simulink model "SWC_HALIN_CDD_type"  (R2021b)
settings: Solver=FixedStepDiscrete  StartTime=0.0  StopTime=10.0  FixedStep=0.005  RelTol=1e-3
undefined symbols (not defined in the file or in its folder): C_TASK_5MS_S, DIDLen_APSFunConfig, DIDLen_AutoLock, DIDLen_AutoWipHSpdEN, DIDLen_DKCKey, DIDLen_DRLDis, DIDLen_DynoMode, DIDLen_FMHTimer, DIDLen_OBDReq, DIDLen_TestGroup, DIDLen_TireSize, DIDLen_TurnLampFLThreCurr, DIDLen_TurnLampFRThreCurr, DIDLen_TurnLampRLThreCurr, DIDLen_TurnLampRRThreCurr, DIDLen_USSConfig, DIDLen_WipRLSCmdCutFilter, DIDLen_WipRLSCmdHoldFilter, DIDLen_XWDMode, DIDNum_APSFunConfig, DIDNum_AutoLock, DIDNum_AutoWipHSpdEN, DIDNum_DKCKey, DIDNum_DRLDis, DIDNum_DynoMode, DIDNum_FMHTimer, DIDNum_OBDReq, DIDNum_TestGroup, DIDNum_TireSize, DIDNum_TurnLampFLThreCurr, DIDNum_TurnLampFRThreCurr, DIDNum_TurnLampRLThreCurr, DIDNum_TurnLampRRThreCurr, DIDNum_USSConfig, DIDNum_WipRLSCmdCutFilter, DIDNum_WipRLSCmdHoldFilter, DIDNum_XWDMode, ENUM_DRIVETRAIN_AWD, ENUM_DRIVETRAIN_FWD, ENUM_DRIVETRAIN_RWD, ENUM_REGENLEVEL_LV1, ENUM_REGENLEVEL_LV2, ENUM_REGENLEVEL_LV3, ENUM_REGENLEVEL_LV4, ENUM_REGENLEVEL_LV5, ENUM_REGENLEVEL_OPD, ENUM_TPMSSTA_FAT, ENUM_TPMSSTA_LOWBATTERY, ENUM_TPMSSTA_TRIGGER, FALSE, FIVE_INT, FOUR_INT, KHAL_CANBusOffDebounce_s, KHAL_DefaultRegenMode_enum, KHAL_DKCDecryptEnable_flg_ovrdflg, KHAL_DKCDecryptEnable_flg_ovrdval, KHAL_RandomNumberY1_enum, KHAL_RandomNumberY2_enum, KHAL_RandomNumberY_ovrdflg, KHAL_TPMSRESBUTT_flg_ovrdflg ... (+9)
libraries: simulink x229, FVT_lib x29, hcu_lib x25, hdlsllib x15
(part 2 of 8)

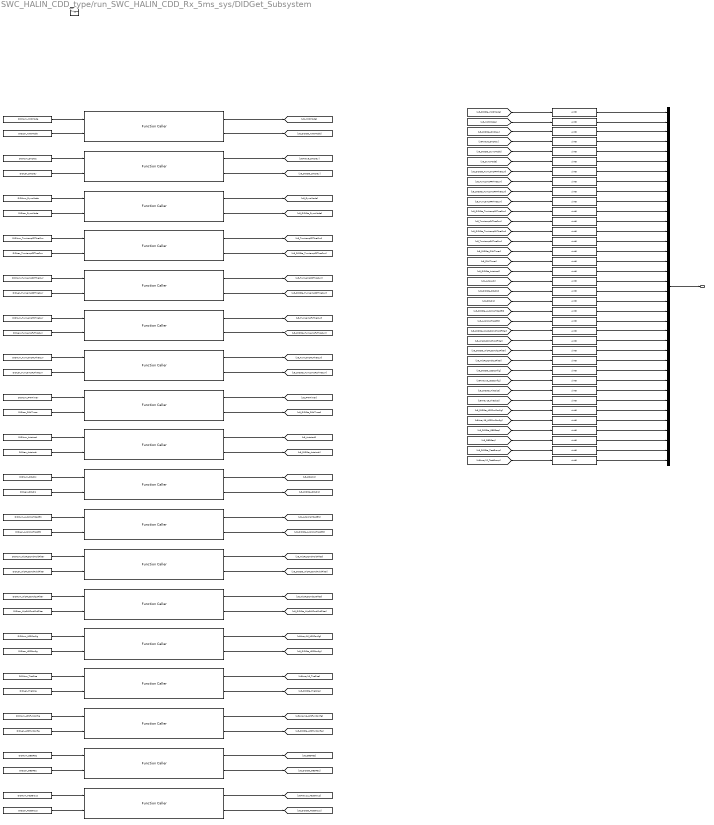
== system SWC_HALIN_CDD_type/run_SWC_HALIN_CDD_Rx_5ms_sys/DIDGet_Subsystem ==
  trig_GetDID : TriggerPort  TriggerType=function-call  VariantControl=(inherit)  PortDimensions=1
  DIDLen : Constant  Value=DIDNum_XWDMode
  DIDLen1 : Constant  Value=DIDNum_DKCKey
  DIDLen10 : Constant  Value=DIDNum_AutoWipHSpdEN
  DIDLen11 : Constant  Value=DIDNum_WipRLSCmdHoldFilter
  DIDLen12 : Constant  Value=DIDNum_WipRLSCmdCutFilter
  DIDLen13 : Constant  Value=DIDNum_USSConfig
  DIDLen14 : Constant  Value=DIDNum_TireSize
  DIDLen15 : Constant  Value=DIDNum_APSFunConfig
  DIDLen16 : Constant  Value=DIDNum_OBDReq
  DIDLen17 : Constant  Value=DIDNum_TestGroup
  DIDLen2 : Constant  Value=DIDNum_DynoMode
  DIDLen3 : Constant  Value=DIDNum_TurnLampFRThreCurr
  DIDLen4 : Constant  Value=DIDNum_TurnLampRRThreCurr
  DIDLen5 : Constant  Value=DIDNum_TurnLampFLThreCurr
  DIDLen6 : Constant  Value=DIDNum_TurnLampRLThreCurr
  DIDLen7 : Constant  Value=DIDNum_FMHTimer
  DIDLen8 : Constant  Value=DIDNum_AutoLock
  DIDLen9 : Constant  Value=DIDNum_DRLDis
  DIDNum : Constant  Value=DIDLen_XWDMode
  DIDNum1 : Constant  Value=DIDLen_DKCKey
  DIDNum10 : Constant  Value=DIDLen_AutoWipHSpdEN
  DIDNum11 : Constant  Value=DIDLen_WipRLSCmdHoldFilter
  DIDNum12 : Constant  Value=DIDLen_WipRLSCmdCutFilter
  DIDNum13 : Constant  Value=DIDLen_USSConfig
  DIDNum14 : Constant  Value=DIDLen_TireSize
  DIDNum15 : Constant  Value=DIDLen_APSFunConfig
  DIDNum16 : Constant  Value=DIDLen_OBDReq
  DIDNum17 : Constant  Value=DIDLen_TestGroup
  DIDNum2 : Constant  Value=DIDLen_DynoMode
  DIDNum3 : Constant  Value=DIDLen_TurnLampFRThreCurr
  DIDNum4 : Constant  Value=DIDLen_TurnLampRRThreCurr
  DIDNum5 : Constant  Value=DIDLen_TurnLampFLThreCurr
  DIDNum6 : Constant  Value=DIDLen_TurnLampRLThreCurr
  DIDNum7 : Constant  Value=DIDLen_FMHTimer
  DIDNum8 : Constant  Value=DIDLen_AutoLock
  DIDNum9 : Constant  Value=DIDLen_DRLDis
  R_DIDReadCDD_CSOP_DIDGet_APSFunConfig : FunctionCaller  FunctionPrototype=[u8Array16_APSFunConfig,u8_DIDSta_APSFunConfig] = R_DIDReadCDD_CSOP_DIDGet_APSFunConfig(u16_DIDNum_APSFunConfig,u16_DIDLen_APSFunConfig)  InputArgumentSpecifications=uint16(1), uint16(1)  OutputArgumentSpecifications=uint8([1;1;1;1;1;1;1;1;1;1;1;1;1;1;1;1]), uint8(1)
  R_DIDReadCDD_CSOP_DIDGet_AutoLock : FunctionCaller  FunctionPrototype=[u8_AutoLock,u8_DIDSta_AutoLock] = R_DIDReadCDD_CSOP_DIDGet_AutoLock(u16_DIDNum_AutoLock,u16_DIDLen_AutoLock)  InputArgumentSpecifications=uint16(1), uint16(1)  OutputArgumentSpecifications=uint8(1), uint8(1)
  R_DIDReadCDD_CSOP_DIDGet_AutoWipHSpdEN : FunctionCaller  FunctionPrototype=[u8_AutoWipHSpdEN,u8_DIDSta_AutoWipHSpdEN] = R_DIDReadCDD_CSOP_DIDGet_AutoWipHSpdEN(u16_DIDNum_AutoWipHSpdEN,u16_DIDLen_AutoWipHSpdEN)  InputArgumentSpecifications=uint16(1), uint16(1)  OutputArgumentSpecifications=uint8(1), uint8(1)
  R_DIDReadCDD_CSOP_DIDGet_DKCKey : FunctionCaller  FunctionPrototype=[u8Array8_DKCKey,u8_DIDSta_DKCKey] = R_DIDReadCDD_CSOP_DIDGet_DKCKey(u16_DIDNum_DKCKey,u16_DIDLen_DKCKey)  InputArgumentSpecifications=uint16(1), uint16(1)  OutputArgumentSpecifications=uint8([1;1;1;1;1;1;1;1]), uint8(1)
  R_DIDReadCDD_CSOP_DIDGet_DRLDis : FunctionCaller  FunctionPrototype=[u8_DRLDis,u8_DIDSta_DRLDis] = R_DIDReadCDD_CSOP_DIDGet_DRLDis(u16_DIDNum_DRLDis,u16_DIDLen_DRLDis)  InputArgumentSpecifications=uint16(1), uint16(1)  OutputArgumentSpecifications=uint8(1), uint8(1)
  R_DIDReadCDD_CSOP_DIDGet_DynoMode : FunctionCaller  FunctionPrototype=[u8_DynoMode,u8_DIDSta_DynoMode] = R_DIDReadCDD_CSOP_DIDGet_DynoMode(u16_DIDNum_DynoMode,u16_DIDLen_DynoMode)  InputArgumentSpecifications=uint16(1), uint16(1)  OutputArgumentSpecifications=uint8(1), uint8(1)
  R_DIDReadCDD_CSOP_DIDGet_FMHTimer : FunctionCaller  FunctionPrototype=[u8_FMHTimer,u8_DIDSta_FMHTimer] = R_DIDReadCDD_CSOP_DIDGet_FMHTimer(u16_DIDNum_FMHTimer,u16_DIDLen_FMHTimer)  InputArgumentSpecifications=uint16(1), uint16(1)  OutputArgumentSpecifications=uint8(1), uint8(1)
  R_DIDReadCDD_CSOP_DIDGet_OBDReq : FunctionCaller  FunctionPrototype=[u8_OBDReq,u8_DIDSta_OBDReq] = R_DIDReadCDD_CSOP_DIDGet_OBDReq(u16_DIDNum_OBDReq,u16_DIDLen_OBDReq)  InputArgumentSpecifications=uint16(1), uint16(1)  OutputArgumentSpecifications=uint8(1), uint8(1)
  R_DIDReadCDD_CSOP_DIDGet_TestGroup : FunctionCaller  FunctionPrototype=[u8Array12_TestGroup,u8_DIDSta_TestGroup] = R_DIDReadCDD_CSOP_DIDGet_TestGroup(u16_DIDNum_TestGroup,u16_DIDLen_TestGroup)  InputArgumentSpecifications=uint16(1), uint16(1)  OutputArgumentSpecifications=uint8([1;1;1;1;1;1;1;1;1;1;1;1]), uint8(1)
  R_DIDReadCDD_CSOP_DIDGet_TireSize : FunctionCaller  FunctionPrototype=[u8Array16_TireSize,u8_DIDSta_TireSize] = R_DIDReadCDD_CSOP_DIDGet_TireSize(u16_DIDNum_TireSize,u16_DIDLen_TireSize)  InputArgumentSpecifications=uint16(1), uint16(1)  OutputArgumentSpecifications=uint8([1;1;1;1;1;1;1;1;1;1;1;1;1;1;1;1]), uint8(1)
  R_DIDReadCDD_CSOP_DIDGet_TurnLampFLThreCurr : FunctionCaller  FunctionPrototype=[u8_TurnLampFLThreCurr,u8_DIDSta_TurnLampFLThreCurr] = R_DIDReadCDD_CSOP_DIDGet_TurnLampFLThreCurr(u16_DIDNum_TurnLampFLThreCurr,u16_DIDLen_TurnLampFLThreCurr)  InputArgumentSpecifications=uint16(1), uint16(1)  OutputArgumentSpecifications=uint8(1), uint8(1)
  R_DIDReadCDD_CSOP_DIDGet_TurnLampFRThreCurr : FunctionCaller  FunctionPrototype=[u8_TurnLampFRThreCurr,u8_DIDSta_TurnLampFRThreCurr] = R_DIDReadCDD_CSOP_DIDGet_TurnLampFRThreCurr(u16_DIDNum_TurnLampFRThreCurr,u16_DIDLen_TurnLampFRThreCurr)  InputArgumentSpecifications=uint16(1), uint16(1)  OutputArgumentSpecifications=uint8(1), uint8(1)
  R_DIDReadCDD_CSOP_DIDGet_TurnLampRLThreCurr : FunctionCaller  FunctionPrototype=[u8_TurnLampRLThreCurr,u8_DIDSta_TurnLampRLThreCurr] = R_DIDReadCDD_CSOP_DIDGet_TurnLampRLThreCurr(u16_DIDNum_TurnLampRLThreCurr,u16_DIDLen_TurnLampRLThreCurr)  InputArgumentSpecifications=uint16(1), uint16(1)  OutputArgumentSpecifications=uint8(1), uint8(1)
  R_DIDReadCDD_CSOP_DIDGet_TurnLampRRThreCurr : FunctionCaller  FunctionPrototype=[u8_TurnLampRRThreCurr,u8_DIDSta_TurnLampRRThreCurr] = R_DIDReadCDD_CSOP_DIDGet_TurnLampRRThreCurr(u16_DIDNum_TurnLampRRThreCurr,u16_DIDLen_TurnLampRRThreCurr)  InputArgumentSpecifications=uint16(1), uint16(1)  OutputArgumentSpecifications=uint8(1), uint8(1)
  R_DIDReadCDD_CSOP_DIDGet_USSConfig : FunctionCaller  FunctionPrototype=[u8Array16_USSConfig,u8_DIDSta_USSConfig] = R_DIDReadCDD_CSOP_DIDGet_USSConfig(u16_DIDNum_USSConfig,u16_DIDLen_USSConfig)  InputArgumentSpecifications=uint16(1), uint16(1)  OutputArgumentSpecifications=uint8([1;1;1;1;1;1;1;1;1;1;1;1;1;1;1;1]), uint8(1)
  R_DIDReadCDD_CSOP_DIDGet_WipRLSCmdCutFilter : FunctionCaller  FunctionPrototype=[u8_WipRLSCmdCutFilter,u8_DIDSta_WipRLSCmdCutFilter] = R_DIDReadCDD_CSOP_DIDGet_WipRLSCmdCutFilter(u16_DIDNum_WipRLSCmdCutFilter,u16_DIDLen_WipRLSCmdCutFilter)  InputArgumentSpecifications=uint16(1), uint16(1)  OutputArgumentSpecifications=uint8(1), uint8(1)
  R_DIDReadCDD_CSOP_DIDGet_WipRLSCmdHoldFilter : FunctionCaller  FunctionPrototype=[u8_WipRLSCmdHoldFilter,u8_DIDSta_WipRLSCmdHoldFilter] = R_DIDReadCDD_CSOP_DIDGet_WipRLSCmdHoldFilter(u16_DIDNum_WipRLSCmdHoldFilter,u16_DIDLen_WipRLSCmdHoldFilter)  InputArgumentSpecifications=uint16(1), uint16(1)  OutputArgumentSpecifications=uint8(1), uint8(1)
  R_DIDReadCDD_CSOP_DIDGet_XWDMode : FunctionCaller  FunctionPrototype=[u8_XWDMode,u8_DIDSta_XWDMode] = R_DIDReadCDD_CSOP_DIDGet_XWDMode(u16_DIDNum_XWDMode,u16_DIDLen_XWDMode)  InputArgumentSpecifications=uint16(1), uint16(1)  OutputArgumentSpecifications=uint8(1), uint8(1)
  UnitConverter{,1..35} (36 alike) : DataTypeConversion  OutDataTypeStr=uint8
  bus_Creator : BusCreator  Inputs=36  OutDataTypeStr=Bus: BHAL_DID_outputs  NonVirtualBus=on
  BHAL_DID_outputs : Outport  OutDataTypeStr=Bus: BHAL_DID_outputs
  wires:
  [u8_DIDSta_XWDMode] -> UnitConverter/1  "u8_DIDSta_XWDMode"
  UnitConverter/1 -> bus_Creator/1  "VHAL_DIDStaXWDMode_raw"
  [u8_XWDMode] -> UnitConverter1/1  "u8_XWDMode"
  UnitConverter1/1 -> bus_Creator/2  "VHAL_XWDMode_raw"
  [u8_DIDSta_DKCKey] -> UnitConverter2/1  "u8_DIDSta_DKCKey"
  UnitConverter2/1 -> bus_Creator/3  "VHAL_DIDStaDKCKey_raw"
  [u8Array8_DKCKey] -> UnitConverter3/1  "u8Array8_DKCKey"
  UnitConverter3/1 -> bus_Creator/4  "VHAL_DKCKey_raw"
  [u8_DIDSta_DynoMode] -> UnitConverter4/1  "u8_DIDSta_DynoMode"
  UnitConverter4/1 -> bus_Creator/5  "VHAL_DIDStaDynoMode_raw"
  [u8_DynoMode] -> UnitConverter5/1  "u8_DynoMode"
  UnitConverter5/1 -> bus_Creator/6  "VHAL_DynoMode_raw"
  [u8_DIDSta_TurnLampFRThreCurr] -> UnitConverter6/1  "u8_DIDSta_TurnLampFRThreCurr"
  UnitConverter6/1 -> bus_Creator/7  "VHAL_DIDStaTurnLampFRThreCurr_raw"
  [u8_TurnLampFRThreCurr] -> UnitConverter7/1  "u8_TurnLampFRThreCurr"
  UnitConverter7/1 -> bus_Creator/8  "VHAL_TurnLampFRThreCurr_raw"
  [u8_DIDSta_TurnLampRRThreCurr] -> UnitConverter8/1  "u8_DIDSta_TurnLampRRThreCurr"
  UnitConverter8/1 -> bus_Creator/9  "VHAL_DIDStaTurnLampRRThreCurr_raw"
  [u8_TurnLampRRThreCurr] -> UnitConverter9/1  "u8_TurnLampRRThreCurr"
  UnitConverter9/1 -> bus_Creator/10  "VHAL_TurnLampRRThreCurr_raw"
  [u8_DIDSta_TurnLampFLThreCurr] -> UnitConverter10/1  "u8_DIDSta_TurnLampFLThreCurr"
  UnitConverter10/1 -> bus_Creator/11  "VHAL_DIDStaTurnLampFLThreCurr_raw"
  [u8_TurnLampFLThreCurr] -> UnitConverter11/1  "u8_TurnLampFLThreCurr"
  UnitConverter11/1 -> bus_Creator/12  "VHAL_TurnLampFLThreCurr_raw"
  [u8_DIDSta_TurnLampRLThreCurr] -> UnitConverter12/1  "u8_DIDSta_TurnLampRLThreCurr"
  UnitConverter12/1 -> bus_Creator/13  "VHAL_DIDStaTurnLampRLThreCurr_raw"
  [u8_TurnLampRLThreCurr] -> UnitConverter13/1  "u8_TurnLampRLThreCurr"
  UnitConverter13/1 -> bus_Creator/14  "VHAL_TurnLampRLThreCurr_raw"
  [u8_DIDSta_FMHTimer] -> UnitConverter14/1  "u8_DIDSta_FMHTimer"
  UnitConverter14/1 -> bus_Creator/15  "VHAL_DIDStaFMHTimer_raw"
  [u8_FMHTimer] -> UnitConverter15/1  "u8_FMHTimer"
  UnitConverter15/1 -> bus_Creator/16  "VHAL_FMHTimer_raw"
  [u8_DIDSta_AutoLock] -> UnitConverter16/1  "u8_DIDSta_AutoLock"
  UnitConverter16/1 -> bus_Creator/17  "VHAL_DIDStaAutoLock_raw"
  [u8_AutoLock] -> UnitConverter17/1  "u8_AutoLock"
  UnitConverter17/1 -> bus_Creator/18  "VHAL_AutoLock_raw"
  [u8_DIDSta_DRLDis] -> UnitConverter18/1  "u8_DIDSta_DRLDis"
  UnitConverter18/1 -> bus_Creator/19  "VHAL_DIDStaDRLDis_raw"
  [u8_DRLDis] -> UnitConverter19/1  "u8_DRLDis"
  UnitConverter19/1 -> bus_Creator/20  "VHAL_DRLDis_raw"
  [u8_DIDSta_AutoWipHSpdEN] -> UnitConverter20/1  "u8_DIDSta_AutoWipHSpdEN"
  UnitConverter20/1 -> bus_Creator/21  "VHAL_DIDStaAutoWipHSpdEN_raw"
  [u8_AutoWipHSpdEN] -> UnitConverter21/1  "u8_AutoWipHSpdEN"
  UnitConverter21/1 -> bus_Creator/22  "VHAL_AutoWipHSpdEN_raw"
  [u8_DIDSta_WipRLSCmdHoldFilter] -> UnitConverter22/1  "u8_DIDSta_WipRLSCmdHoldFilter"
  UnitConverter22/1 -> bus_Creator/23  "VHAL_DIDStaWipRLSCmdHoldFilter_raw"
  [u8_WipRLSCmdHoldFilter] -> UnitConverter23/1  "u8_WipRLSCmdHoldFilter"
  UnitConverter23/1 -> bus_Creator/24  "VHAL_WipRLSCmdHoldFilter_raw"
  [u8_DIDSta_WipRLSCmdCutFilter] -> UnitConverter24/1  "u8_DIDSta_WipRLSCmdCutFilter"
  UnitConverter24/1 -> bus_Creator/25  "VHAL_DIDStaWipRLSCmdCutFilter_raw"
  [u8_WipRLSCmdCutFilter] -> UnitConverter25/1  "u8_WipRLSCmdCutFilter"
  UnitConverter25/1 -> bus_Creator/26  "VHAL_WipRLSCmdCutFilter_raw"
  [u8_DIDSta_USSConfig] -> UnitConverter26/1  "u8_DIDSta_USSConfig"
  UnitConverter26/1 -> bus_Creator/27  "VHAL_DIDStaUSSConfig_raw"
  [u8Array16_USSConfig] -> UnitConverter27/1  "u8Array16_USSConfig"
  UnitConverter27/1 -> bus_Creator/28  "VHAL_USSConfig_raw"
  [u8_DIDSta_TireSize] -> UnitConverter28/1  "u8_DIDSta_TireSize"
  UnitConverter28/1 -> bus_Creator/29  "VHAL_DIDStaTireSize_raw"
  [u8Array16_TireSize] -> UnitConverter29/1  "u8Array16_TireSize"
  UnitConverter29/1 -> bus_Creator/30  "VHAL_TireSize_raw"
  [u8_DIDSta_APSFunConfig] -> UnitConverter30/1  "u8_DIDSta_APSFunConfig"
  UnitConverter30/1 -> bus_Creator/31  "VHAL_DIDStaAPSFunConfig_raw"
  [u8Array16_APSFunConfig] -> UnitConverter31/1  "u8Array16_APSFunConfig"
  UnitConverter31/1 -> bus_Creator/32  "VHAL_APSFunConfig_raw"
  [u8_DIDSta_OBDReq] -> UnitConverter32/1  "u8_DIDSta_OBDReq"
  UnitConverter32/1 -> bus_Creator/33  "VHAL_DIDStaOBDReq_raw"
  [u8_OBDReq] -> UnitConverter33/1  "u8_OBDReq"
  UnitConverter33/1 -> bus_Creator/34  "VHAL_OBDReq_raw"
  [u8_DIDSta_TestGroup] -> UnitConverter34/1  "u8_DIDSta_TestGroup"
  UnitConverter34/1 -> bus_Creator/35  "VHAL_DIDStaTestGroup_raw"
  [u8Array12_TestGroup] -> UnitConverter35/1  "u8Array12_TestGroup"
  UnitConverter35/1 -> bus_Creator/36  "VHAL_TestGroup_raw"
  bus_Creator/1 -> BHAL_DID_outputs/1
  DIDLen/1 -> R_DIDReadCDD_CSOP_DIDGet_XWDMode/1
  DIDNum/1 -> R_DIDReadCDD_CSOP_DIDGet_XWDMode/2
  R_DIDReadCDD_CSOP_DIDGet_XWDMode/1 -> [u8_XWDMode]
  R_DIDReadCDD_CSOP_DIDGet_XWDMode/2 -> [u8_DIDSta_XWDMode]
  DIDLen1/1 -> R_DIDReadCDD_CSOP_DIDGet_DKCKey/1
  DIDNum1/1 -> R_DIDReadCDD_CSOP_DIDGet_DKCKey/2
  R_DIDReadCDD_CSOP_DIDGet_DKCKey/1 -> [u8Array8_DKCKey]
  R_DIDReadCDD_CSOP_DIDGet_DKCKey/2 -> [u8_DIDSta_DKCKey]
  DIDLen2/1 -> R_DIDReadCDD_CSOP_DIDGet_DynoMode/1
  DIDNum2/1 -> R_DIDReadCDD_CSOP_DIDGet_DynoMode/2
  R_DIDReadCDD_CSOP_DIDGet_DynoMode/1 -> [u8_DynoMode]
  R_DIDReadCDD_CSOP_DIDGet_DynoMode/2 -> [u8_DIDSta_DynoMode]
  DIDLen3/1 -> R_DIDReadCDD_CSOP_DIDGet_TurnLampFRThreCurr/1
  DIDNum3/1 -> R_DIDReadCDD_CSOP_DIDGet_TurnLampFRThreCurr/2
  R_DIDReadCDD_CSOP_DIDGet_TurnLampFRThreCurr/1 -> [u8_TurnLampFRThreCurr]
  R_DIDReadCDD_CSOP_DIDGet_TurnLampFRThreCurr/2 -> [u8_DIDSta_TurnLampFRThreCurr]
  DIDLen4/1 -> R_DIDReadCDD_CSOP_DIDGet_TurnLampRRThreCurr/1
  DIDNum4/1 -> R_DIDReadCDD_CSOP_DIDGet_TurnLampRRThreCurr/2
  R_DIDReadCDD_CSOP_DIDGet_TurnLampRRThreCurr/1 -> [u8_TurnLampRRThreCurr]
  R_DIDReadCDD_CSOP_DIDGet_TurnLampRRThreCurr/2 -> [u8_DIDSta_TurnLampRRThreCurr]
  DIDLen5/1 -> R_DIDReadCDD_CSOP_DIDGet_TurnLampFLThreCurr/1
  DIDNum5/1 -> R_DIDReadCDD_CSOP_DIDGet_TurnLampFLThreCurr/2
  R_DIDReadCDD_CSOP_DIDGet_TurnLampFLThreCurr/1 -> [u8_TurnLampFLThreCurr]
  R_DIDReadCDD_CSOP_DIDGet_TurnLampFLThreCurr/2 -> [u8_DIDSta_TurnLampFLThreCurr]
  DIDLen6/1 -> R_DIDReadCDD_CSOP_DIDGet_TurnLampRLThreCurr/1
  DIDNum6/1 -> R_DIDReadCDD_CSOP_DIDGet_TurnLampRLThreCurr/2
  R_DIDReadCDD_CSOP_DIDGet_TurnLampRLThreCurr/1 -> [u8_TurnLampRLThreCurr]
  R_DIDReadCDD_CSOP_DIDGet_TurnLampRLThreCurr/2 -> [u8_DIDSta_TurnLampRLThreCurr]
  DIDLen7/1 -> R_DIDReadCDD_CSOP_DIDGet_FMHTimer/1
  DIDNum7/1 -> R_DIDReadCDD_CSOP_DIDGet_FMHTimer/2
  R_DIDReadCDD_CSOP_DIDGet_FMHTimer/1 -> [u8_FMHTimer]
  R_DIDReadCDD_CSOP_DIDGet_FMHTimer/2 -> [u8_DIDSta_FMHTimer]
  DIDLen8/1 -> R_DIDReadCDD_CSOP_DIDGet_AutoLock/1
  DIDNum8/1 -> R_DIDReadCDD_CSOP_DIDGet_AutoLock/2
  R_DIDReadCDD_CSOP_DIDGet_AutoLock/1 -> [u8_AutoLock]
  R_DIDReadCDD_CSOP_DIDGet_AutoLock/2 -> [u8_DIDSta_AutoLock]
  DIDLen9/1 -> R_DIDReadCDD_CSOP_DIDGet_DRLDis/1
  DIDNum9/1 -> R_DIDReadCDD_CSOP_DIDGet_DRLDis/2
  R_DIDReadCDD_CSOP_DIDGet_DRLDis/1 -> [u8_DRLDis]
  R_DIDReadCDD_CSOP_DIDGet_DRLDis/2 -> [u8_DIDSta_DRLDis]
  DIDLen10/1 -> R_DIDReadCDD_CSOP_DIDGet_AutoWipHSpdEN/1
  DIDNum10/1 -> R_DIDReadCDD_CSOP_DIDGet_AutoWipHSpdEN/2
  R_DIDReadCDD_CSOP_DIDGet_AutoWipHSpdEN/1 -> [u8_AutoWipHSpdEN]
  R_DIDReadCDD_CSOP_DIDGet_AutoWipHSpdEN/2 -> [u8_DIDSta_AutoWipHSpdEN]
  DIDLen11/1 -> R_DIDReadCDD_CSOP_DIDGet_WipRLSCmdHoldFilter/1
  DIDNum11/1 -> R_DIDReadCDD_CSOP_DIDGet_WipRLSCmdHoldFilter/2
  R_DIDReadCDD_CSOP_DIDGet_WipRLSCmdHoldFilter/1 -> [u8_WipRLSCmdHoldFilter]
  R_DIDReadCDD_CSOP_DIDGet_WipRLSCmdHoldFilter/2 -> [u8_DIDSta_WipRLSCmdHoldFilter]
  DIDLen12/1 -> R_DIDReadCDD_CSOP_DIDGet_WipRLSCmdCutFilter/1
  DIDNum12/1 -> R_DIDReadCDD_CSOP_DIDGet_WipRLSCmdCutFilter/2
  R_DIDReadCDD_CSOP_DIDGet_WipRLSCmdCutFilter/1 -> [u8_WipRLSCmdCutFilter]
  R_DIDReadCDD_CSOP_DIDGet_WipRLSCmdCutFilter/2 -> [u8_DIDSta_WipRLSCmdCutFilter]
  DIDLen13/1 -> R_DIDReadCDD_CSOP_DIDGet_USSConfig/1
  DIDNum13/1 -> R_DIDReadCDD_CSOP_DIDGet_USSConfig/2
  R_DIDReadCDD_CSOP_DIDGet_USSConfig/1 -> [u8Array16_USSConfig]
  R_DIDReadCDD_CSOP_DIDGet_USSConfig/2 -> [u8_DIDSta_USSConfig]
  DIDLen14/1 -> R_DIDReadCDD_CSOP_DIDGet_TireSize/1
  DIDNum14/1 -> R_DIDReadCDD_CSOP_DIDGet_TireSize/2
  R_DIDReadCDD_CSOP_DIDGet_TireSize/1 -> [u8Array16_TireSize]
  R_DIDReadCDD_CSOP_DIDGet_TireSize/2 -> [u8_DIDSta_TireSize]
  DIDLen15/1 -> R_DIDReadCDD_CSOP_DIDGet_APSFunConfig/1
  DIDNum15/1 -> R_DIDReadCDD_CSOP_DIDGet_APSFunConfig/2
  R_DIDReadCDD_CSOP_DIDGet_APSFunConfig/1 -> [u8Array16_APSFunConfig]
  R_DIDReadCDD_CSOP_DIDGet_APSFunConfig/2 -> [u8_DIDSta_APSFunConfig]
  DIDLen16/1 -> R_DIDReadCDD_CSOP_DIDGet_OBDReq/1
  DIDNum16/1 -> R_DIDReadCDD_CSOP_DIDGet_OBDReq/2
  R_DIDReadCDD_CSOP_DIDGet_OBDReq/1 -> [u8_OBDReq]
  R_DIDReadCDD_CSOP_DIDGet_OBDReq/2 -> [u8_DIDSta_OBDReq]
  DIDLen17/1 -> R_DIDReadCDD_CSOP_DIDGet_TestGroup/1
  DIDNum17/1 -> R_DIDReadCDD_CSOP_DIDGet_TestGroup/2
  R_DIDReadCDD_CSOP_DIDGet_TestGroup/1 -> [u8Array12_TestGroup]
  R_DIDReadCDD_CSOP_DIDGet_TestGroup/2 -> [u8_DIDSta_TestGroup]

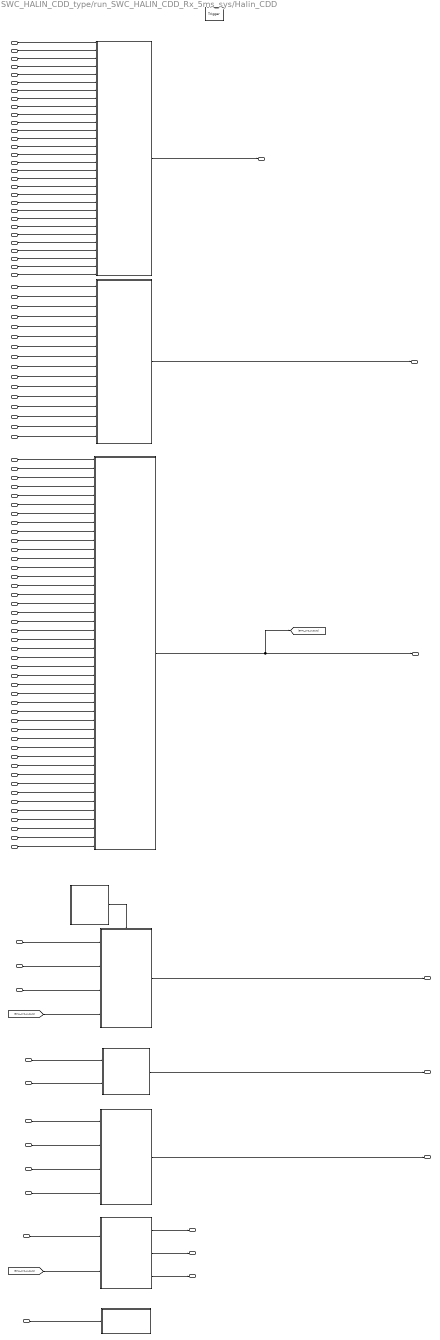
== system SWC_HALIN_CDD_type/run_SWC_HALIN_CDD_Rx_5ms_sys/Halin_CDD ==
  PASDistanceData : Inport
  APSDistanceData : Inport  Port=2
  APSLevelData : Inport  Port=3
  APSFaultStaData : Inport  Port=4
  ChimeIn : Inport  Port=5
  SNSRLayoutIn : Inport  Port=6
  StaFSyaIn : Inport  Port=7
  ModOperationIn : Inport  Port=8
  VHAL_AccelPedal1Vol_Raw : Inport  Port=9
  VHAL_AccelPedal2Vol_Raw : Inport  Port=10
  VHAL_BrakeSWGPIO_flg : Inport  Port=11
  VHAL_HoodSW_flg : Inport  Port=12
  VHAL_TailgateSW_flg : Inport  Port=13
  VHAL_DrDoorSW_flg : Inport  Port=14
  VHAL_PsDoorSW_flg : Inport  Port=15
  VHAL_RRDoorSW_flg : Inport  Port=16
  VHAL_RLDoorSW_flg : Inport  Port=17
  VHAL_CentralDoorLockSW_flg : Inport  Port=18
  VHAL_HazardSW_flg : Inport  Port=19
  VHAL_BrakeLampSW_flg : Inport  Port=20
  VHAL_TrunkHanSW_flg : Inport  Port=21
  VHAL_SeatSW_flg : Inport  Port=22
  VHAL_CrashSignalGPIO_flg : Inport  Port=23
  u8_HWID_4byte : Inport  Port=24
  GetSWID_status : Inport  Port=25
  GetSWID_data : Inport  Port=26
  VHAL_AnyNMID_flg : Inport  Port=27
  VHAL_CurrentNmState_enum : Inport  Port=28
  VHAL_PwrReq_OTA_enum : Inport  Port=29
  VHAL_AllowMovThd_OTA_enum : Inport  Port=30
  VHAL_EvccAplusPwrUpReq_flg : Inport  Port=31
  VHAL_AcoreReadyToSlp_flg : Inport  Port=32
  VHAL_DidXWDSta_flg : Inport  Port=33
  VHAL_DidXWDData_enum : Inport  Port=34
  HAL_NvmReadData_raw : Inport  Port=35
  VHAL_DIDVCUKeyReadSta_flg : Inport  Port=36
  VHAL_GetDIDVCUKey_enum : Inport  Port=37
  TPMS_DataIn_flg : Inport  Port=38
  TPMS_RawData : Inport  Port=39
  BHAL_CAN2_outputs : Inport  Port=40
  BHAL_CAN4_outputs : Inport  Port=41
  VHAL_ClearDTCcmd_flg : Inport  Port=42
  VHAL_IMUOffsetVal_raw : Inport  Port=43
  VHAL_IMUSixAxisVal_raw : Inport  Port=44
  VHAL_IMUOffsetValSta_flg : Inport  Port=45
  VHAL_IMUSixAxisValSta_flg : Inport  Port=46
  VHAL_NvmProtectSta_flg : Inport  Port=47
  VHAL_AuxBattVolmV_100mV : Inport  Port=48
  VHAL_Pedal1Ref5V_raw : Inport  Port=49
  VHAL_Pedal2Ref5V_raw : Inport  Port=50
  VHAL_NetworkReqCalled_flg : Inport  Port=51
  VHAL_PmicBootReason_enum : Inport  Port=52
  VHAL_WisrBootReason_raw32 : Inport  Port=53
  BHAL_DIDGetData_raw : Inport  Port=54
  VHAL_AcoreRebootCmd_raw : Inport  Port=55
  VHAL_CAN1BusOff_raw : Inport  Port=56
  VHAL_CAN2BusOff_raw : Inport  Port=57
  VHAL_CAN3BusOff_raw : Inport  Port=58
  VHAL_CAN4BusOff_raw : Inport  Port=59
  VHAL_CAN5BusOff_raw : Inport  Port=60
  VHAL_CAN6BusOff_raw : Inport  Port=61
  u8_GetAPS_Progress_PCT : Inport  Port=62
  u8_GetAPS_RQ_Display : Inport  Port=63
  u8_GetAPS_SW_Ver : Inport  Port=64
  u8_GetAPS_HW_Ver : Inport  Port=65
  u8_GetAPS_ExitCondition : Inport  Port=66
  f32_GetAPS_Angle_Target : Inport  Port=67
  u8_GetAPS_Sta_System : Inport  Port=68
  u8_GetAPS_V_Rq_EPAS_Ctrl : Inport  Port=69
  u8_GetAPS_Rq_EPAS_Ctrl : Inport  Port=70
  u8_GetAPS_Req : Inport  Port=71
  f32_GetAPS_DecReq : Inport  Port=72
  u8_GetAPS_DecReq_A : Inport  Port=73
  f32_GetAPS_SpeedCmd : Inport  Port=74
  u8_GetAPS_ShftPosnReq : Inport  Port=75
  u8_GetAPS_VMC_Req_A : Inport  Port=76
  u8_GetCAAS_Sta : Inport  Port=77
  u8_GetCAAS_VMC_Req_A : Inport  Port=78
  u8_GetAPS_PwrReq_cmd : Inport  Port=79
  u8_GetRAPS_BCM_LockReq_Cmd : Inport  Port=80
  u8_GetRAPS_BCM_Lamp_Cmd : Inport  Port=81
  u8_GetRAPS_ErrWarn_Sta : Inport  Port=82
  u8_GetRAPS_ErrLv1_flg : Inport  Port=83
  u8_TPMSSensorIDRegSta : Inport  Port=84
  u8_ResetPedalZeroPosReq : Inport  Port=85
  u32_BootPath : Inport  Port=86
  u8Array17_VinCode : Inport  Port=87
  R_CAN5_FD5_CONN1 : Inport  Port=88
  VHAL_CAN1RxErrorCount_raw : Inport  Port=89
  VHAL_CAN1TxErrorCount_raw : Inport  Port=90
  VHAL_CAN2RxErrorCount_raw : Inport  Port=91
  VHAL_CAN2TxErrorCount_raw : Inport  Port=92
  VHAL_CAN3RxErrorCount_cnt : Inport  Port=93
  VHAL_CAN3TxErrorCount_raw : Inport  Port=94
  VHAL_CAN4RxErrorCount_raw : Inport  Port=95
  VHAL_CAN4TxErrorCount_raw : Inport  Port=96
  VHAL_CAN5RxErrorCount_raw : Inport  Port=97
  VHAL_CAN5TxErrorCount_raw : Inport  Port=98
  VHAL_CAN6RxErrorCount_raw : Inport  Port=99
  VHAL_CAN6TxErrorCount_raw : Inport  Port=100
  VHAL_ClearZevDTCcmd_flg : Inport  Port=101
  trig_HalinCDD : TriggerPort  TriggerType=function-call  VariantControl=(inherit)
  Halin_APM : Subsystem
  Halin_DKC_A : Subsystem
  Halin_GPIO : Subsystem
  Halin_IMU : Subsystem
  Halin_SYS : Subsystem
  Halin_TPMS : Subsystem
  Subsystem : Subsystem
  Subsystem7 : Subsystem
  TPM_Scheduler : Stateflow chart  TreatAsAtomicUnit=on
  BHAL_APM_outputs : Outport
  BHAL_GPIO_outputs : Outport  Port=2
  BHAL_SYS_outputs : Outport  Port=3
  BHAL_TPMS_outputs : Outport  Port=4
  BHAL_DDM_outputs : Outport  Port=5
  BHAL_IMU_outputs : Outport  Port=6
  Enable_decrypt : Outport  Port=7
  AESKey : Outport  Port=8
  DKCRawData : Outport  Port=9
  wires:
  Halin_DKC_A/1(Enable_Decrypt) -> Enable_decrypt/1
  VHAL_RLDoorSW_flg/1 -> Halin_GPIO/9(VHAL_RLDoorSW_flg)
  Halin_SYS/1(BHAL_SYS_outputs) -> [BHAL_SYS_outputs], BHAL_SYS_outputs/1
  Halin_DKC_A/3(DKCRawData) -> DKCRawData/1
  GetSWID_data/1 -> Halin_SYS/2(GetSWID_data)
  VHAL_GetDIDVCUKey_enum/1 -> Halin_SYS/13(VHAL_GetDIDVCUKey_enum)
  VHAL_TailgateSW_flg/1 -> Halin_GPIO/5(VHAL_TailgateSW_flg)
  Halin_DKC_A/2(AESKey) -> AESKey/1
  VHAL_AccelPedal2Vol_Raw/1 -> Halin_GPIO/2(VHAL_AccelPedal2Vol_Raw)
  TPM_Scheduler/1(trig_TPM_10ms1()) -> Halin_TPMS/Trigger
  VHAL_TrunkHanSW_flg/1 -> Halin_GPIO/13(VHAL_TrunkHanSW_flg)
  VHAL_DidXWDSta_flg/1 -> Halin_SYS/9(VHAL_DidXWDSta_flg)
  VHAL_CurrentNmState_enum/1 -> Halin_SYS/4(VHAL_CurrentNmState_enum)
  VHAL_AccelPedal1Vol_Raw/1 -> Halin_GPIO/1(VHAL_AccelPedal1Vol_Raw)
  u8_HWID_4byte/1 -> Halin_GPIO/16(u8_HWID_4byte)
  BHAL_CAN2_outputs/1 -> Halin_TPMS/3(BHAL_CAN2_outputs)
  VHAL_AcoreReadyToSlp_flg/1 -> Halin_SYS/8(VHAL_AcoreReadyToSlp_flg)
  HAL_NvmReadData_raw/1 -> Halin_SYS/11(HAL_NvmReadData_raw)
  VHAL_AllowMovThd_OTA_enum/1 -> Halin_SYS/6(VHAL_AllowMovThd_OTA_enum)
  VHAL_BrakeLampSW_flg/1 -> Halin_GPIO/12(VHAL_BrakeLampSW_flg)
  VHAL_RRDoorSW_flg/1 -> Halin_GPIO/8(VHAL_RRDoorSW_flg)
  VHAL_BrakeSWGPIO_flg/1 -> Halin_GPIO/3(VHAL_BrakeSWGPIO_flg)
  GetSWID_status/1 -> Halin_SYS/1(GetSWID_status)
  VHAL_DrDoorSW_flg/1 -> Halin_GPIO/6(VHAL_DrDoorSW_flg)
  VHAL_PwrReq_OTA_enum/1 -> Halin_SYS/5(VHAL_PwrReq_OTA_enum)
  VHAL_HoodSW_flg/1 -> Halin_GPIO/4(VHAL_HoodSW_flg)
  Halin_GPIO/1(BHAL_GPIO_outputs) -> BHAL_GPIO_outputs/1
  BHAL_CAN4_outputs/1 -> Halin_DKC_A/1(BHAL_CAN4_outputs)
  VHAL_CentralDoorLockSW_flg/1 -> Halin_GPIO/10(VHAL_CentralDoorLockSW_flg)
  TPMS_RawData/1 -> Halin_TPMS/2(TPMS_RawData)
  VHAL_CrashSignalGPIO_flg/1 -> Halin_GPIO/15(VHAL_CrashSignalGPIO_flg)
  Halin_TPMS/1(BHAL_TPMS_outputs) -> BHAL_TPMS_outputs/1
  VHAL_DidXWDData_enum/1 -> Halin_SYS/10(VHAL_DidXWDData_enum)
  VHAL_EvccAplusPwrUpReq_flg/1 -> Halin_SYS/7(VHAL_EvccAplusPwrUpReq_flg)
  VHAL_SeatSW_flg/1 -> Halin_GPIO/14(VHAL_SeatSW_flg)
  VHAL_DIDVCUKeyReadSta_flg/1 -> Halin_SYS/12(VHAL_DIDVCUKeyReadSta_flg)
  VHAL_PsDoorSW_flg/1 -> Halin_GPIO/7(VHAL_PsDoorSW_flg)
  [BHAL_SYS_outputs] -> Halin_DKC_A/2(BHAL_SYS_outputs)
  TPMS_DataIn_flg/1 -> Halin_TPMS/1(TPMS_DataIn_flg)
  VHAL_AnyNMID_flg/1 -> Halin_SYS/3(VHAL_AnyNMID_flg)
  VHAL_HazardSW_flg/1 -> Halin_GPIO/11(VHAL_HazardSW_flg)
  [BHAL_SYS_outputs] -> Halin_TPMS/4(BHAL_SYSTPMS_outputs)
  VHAL_ClearDTCcmd_flg/1 -> Subsystem/1(VHAL_ClearDTCcmd_flg)
  Subsystem/1(BHAL_DDM_outputs) -> BHAL_DDM_outputs/1
  Halin_IMU/1(BHAL_IMU_outputs) -> BHAL_IMU_outputs/1
  VHAL_IMUOffsetVal_raw/1 -> Halin_IMU/1(VHAL_IMUOffsetVal_raw)
  VHAL_IMUOffsetValSta_flg/1 -> Halin_IMU/3(VHAL_IMUOffsetValSta_flg)
  VHAL_IMUSixAxisVal_raw/1 -> Halin_IMU/2(VHAL_IMUSixAxisVal_raw)
  VHAL_IMUSixAxisValSta_flg/1 -> Halin_IMU/4(VHAL_IMUSixAxisValSta_flg)
  VHAL_NvmProtectSta_flg/1 -> Halin_SYS/14(VHAL_NvmProtectSta_flg)
  VHAL_AuxBattVolmV_100mV/1 -> Halin_SYS/15(VHAL_AuxBattVolmV_100mV)
  VHAL_Pedal1Ref5V_raw/1 -> Halin_SYS/16(VHAL_Pedal1Ref5V_raw)
  VHAL_Pedal2Ref5V_raw/1 -> Halin_SYS/17(VHAL_Pedal2Ref5V_raw)
  VHAL_NetworkReqCalled_flg/1 -> Halin_SYS/18(VHAL_NetworkReqCalled_flg)
  VHAL_PmicBootReason_enum/1 -> Halin_SYS/19(VHAL_PmicBootReason_enum)
  VHAL_WisrBootReason_raw32/1 -> Halin_SYS/20(VHAL_WisrBootReason_raw32)
  BHAL_DIDGetData_raw/1 -> Halin_SYS/21(BHAL_DIDGetData_raw)
  VHAL_AcoreRebootCmd_raw/1 -> Halin_SYS/22(VHAL_AcoreRebootCmd_raw)
  VHAL_CAN1BusOff_raw/1 -> Halin_SYS/23(VHAL_CAN1BusOff_raw)
  VHAL_CAN2BusOff_raw/1 -> Halin_SYS/24(VHAL_CAN2BusOff_raw)
  VHAL_CAN3BusOff_raw/1 -> Halin_SYS/25(VHAL_CAN3BusOff_raw)
  VHAL_CAN4BusOff_raw/1 -> Halin_SYS/26(VHAL_CAN4BusOff_raw)
  VHAL_CAN5BusOff_raw/1 -> Halin_SYS/27(VHAL_CAN5BusOff_raw)
  PASDistanceData/1 -> Halin_APM/1(PASDistanceData)
  APSDistanceData/1 -> Halin_APM/2(APSDistanceData)
  APSLevelData/1 -> Halin_APM/3(APSLevelData)
  APSFaultStaData/1 -> Halin_APM/4(APSFaultStaData)
  ChimeIn/1 -> Halin_APM/5(ChimeIn)
  SNSRLayoutIn/1 -> Halin_APM/6(SNSRLayoutIn)
  StaFSyaIn/1 -> Halin_APM/7(StaFSyaIn)
  ModOperationIn/1 -> Halin_APM/8(ModOperationIn)
  u8_GetAPS_Progress_PCT/1 -> Halin_APM/9(u8_GetAPS_Progress_PCT)
  u8_GetAPS_RQ_Display/1 -> Halin_APM/10(u8_GetAPS_RQ_Display)
  u8_GetAPS_SW_Ver/1 -> Halin_APM/11(u8_GetAPS_SW_Ver)
  u8_GetAPS_HW_Ver/1 -> Halin_APM/12(u8_GetAPS_HW_Ver)
  u8_GetAPS_ExitCondition/1 -> Halin_APM/13(u8_GetAPS_ExitCondition)
  f32_GetAPS_Angle_Target/1 -> Halin_APM/14(f32_GetAPS_Angle_Target)
  u8_GetAPS_Sta_System/1 -> Halin_APM/15(u8_GetAPS_Sta_System)
  u8_GetAPS_V_Rq_EPAS_Ctrl/1 -> Halin_APM/16(u8_GetAPS_V_Rq_EPAS_Ctrl)
  u8_GetAPS_Rq_EPAS_Ctrl/1 -> Halin_APM/17(u8_GetAPS_Rq_EPAS_Ctrl)
  u8_GetAPS_Req/1 -> Halin_APM/18(u8_GetAPS_Req)
  f32_GetAPS_DecReq/1 -> Halin_APM/19(f32_GetAPS_DecReq)
  u8_GetAPS_DecReq_A/1 -> Halin_APM/20(u8_GetAPS_DecReq_A)
  f32_GetAPS_SpeedCmd/1 -> Halin_APM/21(f32_GetAPS_SpeedCmd)
  u8_GetAPS_ShftPosnReq/1 -> Halin_APM/22(u8_GetAPS_ShftPosnReq)
  u8_GetAPS_VMC_Req_A/1 -> Halin_APM/23(u8_GetAPS_VMC_Req_A)
  u8_GetCAAS_Sta/1 -> Halin_APM/24(u8_GetCAAS_Sta)
  u8_GetCAAS_VMC_Req_A/1 -> Halin_APM/25(u8_GetCAAS_VMC_Req_A)
  u8_GetAPS_PwrReq_cmd/1 -> Halin_APM/26(u8_GetAPS_PwrReq_cmd)
  u8_GetRAPS_BCM_LockReq_Cmd/1 -> Halin_APM/27(u8_GetRAPS_BCM_LockReq_Cmd)
  u8_GetRAPS_BCM_Lamp_Cmd/1 -> Halin_APM/28(u8_GetRAPS_BCM_Lamp_Cmd)
  u8_GetRAPS_ErrWarn_Sta/1 -> Halin_APM/29(u8_GetRAPS_ErrWarn_Sta)
  u8_GetRAPS_ErrLv1_flg/1 -> Halin_APM/30(u8_GetRAPS_ErrLv1_flg)
  Halin_APM/1(BHAL_APM_outputs) -> BHAL_APM_outputs/1
  u8_TPMSSensorIDRegSta/1 -> Halin_SYS/29(u8_TPMSSensorIDRegSta)
  u8_ResetPedalZeroPosReq/1 -> Halin_SYS/30(VHAL_ResetPedalZeroPosReq_raw)
  VHAL_CAN6BusOff_raw/1 -> Halin_SYS/28(VHAL_CAN6BusOff_raw)
  u32_BootPath/1 -> Halin_SYS/31(VHAL_PmicBootPath_raw32)
  u8Array17_VinCode/1 -> Subsystem7/1(u8Array17_VinCode)
  R_CAN5_FD5_CONN1/1 -> Halin_SYS/32(R_CAN5_FD5_CONN1)
  VHAL_CAN5TxErrorCount_raw/1 -> Halin_SYS/42(VHAL_CAN5TxErrorCount_raw)
  VHAL_CAN6RxErrorCount_raw/1 -> Halin_SYS/43(VHAL_CAN6RxErrorCount_raw)
  VHAL_CAN4TxErrorCount_raw/1 -> Halin_SYS/40(VHAL_CAN4TxErrorCount_raw)
  VHAL_CAN4RxErrorCount_raw/1 -> Halin_SYS/39(VHAL_CAN4RxErrorCount_raw)
  VHAL_CAN3TxErrorCount_raw/1 -> Halin_SYS/38(VHAL_CAN3TxErrorCount_raw)
  VHAL_CAN3RxErrorCount_cnt/1 -> Halin_SYS/37(VHAL_CAN3RxErrorCount_raw)
  VHAL_CAN2TxErrorCount_raw/1 -> Halin_SYS/36(VHAL_CAN2TxErrorCount_raw)
  VHAL_CAN2RxErrorCount_raw/1 -> Halin_SYS/35(VHAL_CAN2RxErrorCount_raw)
  VHAL_CAN6TxErrorCount_raw/1 -> Halin_SYS/44(VHAL_CAN6TxErrorCount_raw)
  VHAL_CAN1TxErrorCount_raw/1 -> Halin_SYS/34(VHAL_CAN1TxErrorCount_raw)
  VHAL_CAN5RxErrorCount_raw/1 -> Halin_SYS/41(VHAL_CAN5RxErrorCount_raw)
  VHAL_CAN1RxErrorCount_raw/1 -> Halin_SYS/33(VHAL_CAN1RxErrorCount_raw)
  VHAL_ClearZevDTCcmd_flg/1 -> Subsystem/2(VHAL_ClearZevDTCcmd_flg)

== system SWC_HALIN_CDD_type/run_SWC_HALIN_CDD_Rx_5ms_sys/R_HALINCDD_CSOP_GetVinCode ==
  Enable : EnablePort
  R_HALINCDD_CSOP_GetVinCode : FunctionCaller  FunctionPrototype=u8Array17_VinCode = R_HALINCDD_CSOP_GetVinCode()  OutputArgumentSpecifications=uint8([1;1;1;1;1;1;1;1;1;1;1;1;1;1;1;1;1])
  Out1 : Outport
  wires:
  R_HALINCDD_CSOP_GetVinCode/1 -> Out1/1

== system SWC_HALIN_CDD_type/run_SWC_HALIN_CDD_Rx_5ms_sys/R_HALIN_IMU_CSOP_IMUGetOffsetVal ==
  trig_ReadIMUOffset_00 : TriggerPort  TriggerType=function-call  VariantControl=(inherit)  PortDimensions=1
  R_HALIN_IMU_CSOP_IMUGetOffsetVal : FunctionCaller  FunctionPrototype=[s16_IMUOffsetVal,u8_IMUOffsetValSta] = R_HALIN_IMU_CSOP_IMUGetOffsetVal()  OutputArgumentSpecifications=int16([1;1;1;1;1;1]), uint8(1)
  Out1 : Outport
  Out2 : Outport  Port=2
  wires:
  R_HALIN_IMU_CSOP_IMUGetOffsetVal/1 -> Out1/1
  R_HALIN_IMU_CSOP_IMUGetOffsetVal/2 -> Out2/1

== system SWC_HALIN_CDD_type/run_SWC_HALIN_CDD_Rx_5ms_sys/Subsystem ==
  Enable_Decrypt : Inport
  AESKey : Inport  Port=2
  DKCRawData : Inport  Port=3
  BHAL_CAN4_outputs : Inport  Port=4
  u8Array3_DKCData : Inport  Port=5
  u8_DKCButton : Inport  Port=6
  u8_DKCUIDBLEStatus : Inport  Port=7
  u8Array2_DKCUIDBLEVol : Inport  Port=8
  s8_DKCUIDBLERSSI : Inport  Port=9
  u8Array10_UWBDistanceCM : Inport  Port=10
  s8Array5_UWBPowerdB : Inport  Port=11
  s8Array2_UWBpositionXCM : Inport  Port=12
  s8Array2_UWBpositionYCM : Inport  Port=13
  u8Array5_UWBRangingSta : Inport  Port=14
  u8_UWBStaRangingONOFF : Inport  Port=15
  function : TriggerPort  TriggerType=function-call  VariantControl=(inherit)
  DKC2 : Subsystem
  R_HALINCDD_CSOP_DKCDecrypt : FunctionCaller  FunctionPrototype=u8Array16_ResultData = R_HALINCDD_CSOP_DKCDecrypt(u8Array16_AESkey,u8Array16_RawData)  InputArgumentSpecifications=uint8([1;1;1;1;1;1;1;1;1;1;1;1;1;1;1;1]), uint8([1;1;1;1;1;1;1;1;1;1;1;1;1;1;1;1])  OutputArgumentSpecifications=uint8([1;1;1;1;1;1;1;1;1;1;1;1;1;1;1;1])
  BHAL_DKC_outputs : Outport
  wires:
  u8Array5_UWBRangingSta/1 -> DKC2/13(u8Array5_UWBRangingSta)
  BHAL_CAN4_outputs/1 -> DKC2/3(BHAL_CAN4_outputs)
  R_HALINCDD_CSOP_DKCDecrypt/1 -> DKC2/2(DKC_ResultData_16byte)
  Enable_Decrypt/1 -> DKC2/1(Enable_Decrypt)
  s8Array2_UWBpositionYCM/1 -> DKC2/12(s8Array2_UWBpositionYCM)
  u8Array10_UWBDistanceCM/1 -> DKC2/9(u8Array10_UWBDistanceCM)
  u8_DKCUIDBLEStatus/1 -> DKC2/6(u8_DKCUIDBLEStatus)
  AESKey/1 -> R_HALINCDD_CSOP_DKCDecrypt/1
  DKC2/1(BHAL_DKC_outputs) -> BHAL_DKC_outputs/1
  u8Array2_DKCUIDBLEVol/1 -> DKC2/7(u8Array2_DKCUIDBLEVol)
  DKCRawData/1 -> R_HALINCDD_CSOP_DKCDecrypt/2
  s8Array5_UWBPowerdB/1 -> DKC2/10(s8Array5_UWBPowerdB)
  u8Array3_DKCData/1 -> DKC2/4(u8Array3_DKCData)
  u8_DKCButton/1 -> DKC2/5(u8_DKCButton)
  s8Array2_UWBpositionXCM/1 -> DKC2/11(s8Array2_UWBpositionXCM)
  s8_DKCUIDBLERSSI/1 -> DKC2/8(s8_DKCUIDBLERSSI)
  u8_UWBStaRangingONOFF/1 -> DKC2/14(u8_UWBStaRangingONOFF)

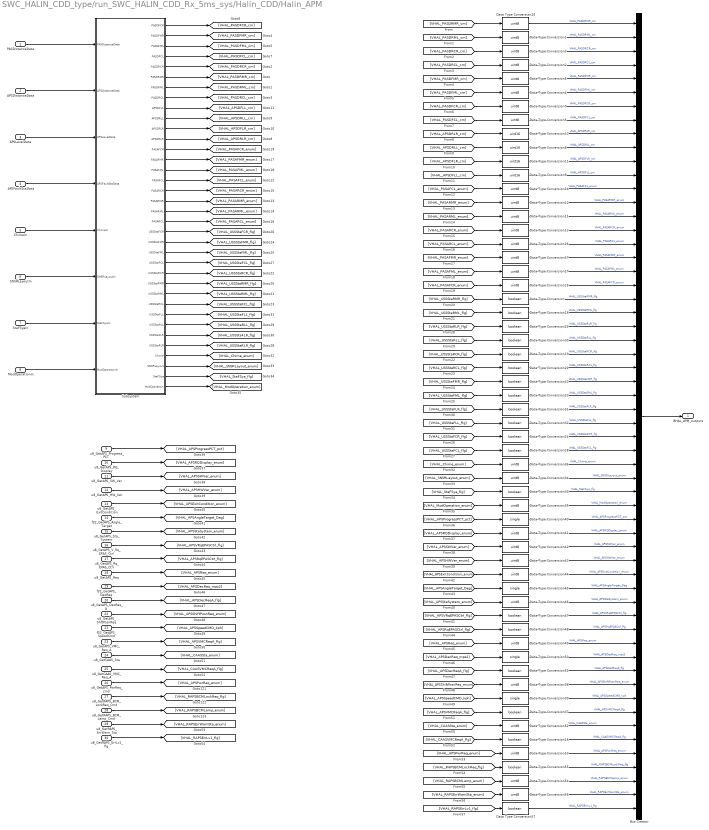
== system SWC_HALIN_CDD_type/run_SWC_HALIN_CDD_Rx_5ms_sys/Halin_CDD/Halin_APM ==
  PASDistanceData : Inport
  APSDistanceData : Inport  Port=2
  APSLevelData : Inport  Port=3
  APSFaultStaData : Inport  Port=4
  ChimeIn : Inport  Port=5
  SNSRLayoutIn : Inport  Port=6
  StaFSyaIn : Inport  Port=7
  ModOperationIn : Inport  Port=8
  u8_GetAPS_Progress_PCT : Inport  Port=9
  u8_GetAPS_RQ_Display : Inport  Port=10
  u8_GetAPS_SW_Ver : Inport  Port=11
  u8_GetAPS_HW_Ver : Inport  Port=12
  u8_GetAPS_ExitCondition : Inport  Port=13
  f32_GetAPS_Angle_Target : Inport  Port=14
  u8_GetAPS_Sta_System : Inport  Port=15
  u8_GetAPS_V_Rq_EPAS_Ctrl : Inport  Port=16
  u8_GetAPS_Rq_EPAS_Ctrl : Inport  Port=17
  u8_GetAPS_Req : Inport  Port=18
  f32_GetAPS_DecReq : Inport  Port=19
  u8_GetAPS_DecReq_A : Inport  Port=20
  f32_GetAPS_SpeedCmd : Inport  Port=21
  u8_GetAPS_ShftPosnReq : Inport  Port=22
  u8_GetAPS_VMC_Req_A : Inport  Port=23
  u8_GetCAAS_Sta : Inport  Port=24
  u8_GetCAAS_VMC_Req_A : Inport  Port=25
  u8_GetAPS_PwrReq_cmd : Inport  Port=26
  u8_GetRAPS_BCM_LockReq_Cmd : Inport  Port=27
  u8_GetRAPS_BCM_Lamp_Cmd : Inport  Port=28
  u8_GetRAPS_ErrWarn_Sta : Inport  Port=29
  u8_GetRAPS_ErrLv1_flg : Inport  Port=30
  Bus Creator : BusCreator  Inputs=58  OutDataTypeStr=Bus: BHAL_APM_outputs  NonVirtualBus=on
  Data Type Conversion{,16,18..19,21..24,28..33,37,47..48,51,55,57} (20 alike) : DataTypeConversion  OutDataTypeStr=boolean
  Data Type Conversion{1..7,12..15,17,20,25..27,34..36,38,41..44,46,49,52..54,56} (30 alike) : DataTypeConversion  OutDataTypeStr=uint8
  Data Type Conversion{8..11} (4 alike) : DataTypeConversion  OutDataTypeStr=uint16
  Data Type Conversion{39..40,45,50} (4 alike) : DataTypeConversion  OutDataTypeStr=single
  Subsystem : Subsystem
  BHAL_APM_outputs : Outport
  wires:
  [VHAL_USSStaRMR_flg] -> Data Type Conversion/1
  Data Type Conversion4/1 -> Bus Creator/6  "VHAL_PASDFML_cm"
  Subsystem/11(APSDFLR) -> [VHAL_APSDFLR_cm]
  [VHAL_PASARCL_enum] -> Data Type Conversion26/1
  Subsystem/36(ModOperation) -> [VHAL_ModOperation_enum]
  Bus Creator/1 -> BHAL_APM_outputs/1
  [VHAL_PASDRCR_cm] -> Data Type Conversion3/1
  [VHAL_PASDRML_cm] -> Data Type Conversion1/1
  Data Type Conversion15/1 -> Bus Creator/15  "VHAL_PASARML_enum"
  [VHAL_USSStaFCR_flg] -> Data Type Conversion24/1
  [VHAL_SNSRLayout_enum] -> Data Type Conversion34/1
  Subsystem/12(APSDRLR) -> [VHAL_APSDRLR_cm]
  Data Type Conversion3/1 -> Bus Creator/3  "VHAL_PASDRCR_cm"
  [VHAL_APSDRLR_cm] -> Data Type Conversion10/1
  Data Type Conversion12/1 -> Bus Creator/14  "VHAL_PASARMR_enum"
  Data Type Conversion33/1 -> Bus Creator/35  "VHAL_StaFSya_flg"
  [VHAL_PASARCR_enum] -> Data Type Conversion13/1
  Subsystem/9(APSDFLL) -> [VHAL_APSDFLL_cm]
  [VHAL_StaFSya_flg] -> Data Type Conversion33/1
  [VHAL_USSStaRLL_flg] -> Data Type Conversion30/1
  Subsystem/4(PASDFCL) -> [VHAL_PASDFCL_cm]
  Subsystem/35(StaFSya) -> [VHAL_StaFSya_flg]
  Subsystem/20(PASARCL) -> [VHAL_PASARCL_enum]
  [VHAL_PASDFML_cm] -> Data Type Conversion4/1
  [VHAL_PASDRMR_cm] -> Data Type Conversion20/1
  Subsystem/16(PASAFCL) -> [VHAL_PASAFCL_enum]
  [VHAL_USSStaFCL_flg] -> Data Type Conversion28/1
  Subsystem/18(PASARMR) -> [VHAL_PASARMR_enum]
  Data Type Conversion13/1 -> Bus Creator/16  "VHAL_PASARCR_enum"
  [VHAL_PASARML_enum] -> Data Type Conversion15/1
  [VHAL_APSDFLL_cm] -> Data Type Conversion9/1
  Subsystem/15(PASAFML) -> [VHAL_PASAFML_enum]
  [VHAL_USSStaFLL_flg] -> Data Type Conversion32/1
  Subsystem/8(PASDRCL) -> [VHAL_PASDRCL_cm]
  Subsystem/27(USSStaRML) -> [VHAL_USSStaRML_flg]
  Data Type Conversion6/1 -> Bus Creator/5  "VHAL_PASDFMR_cm"
  [VHAL_PASAFMR_enum] -> Data Type Conversion17/1
  Data Type Conversion28/1 -> Bus Creator/32  "VHAL_USSStaFCL_flg"
  Subsystem/3(PASDFML) -> [VHAL_PASDFML_cm]
  Data Type Conversion9/1 -> Bus Creator/12  "VHAL_APSDFLL_cm"
  Subsystem/24(USSStaFCL) -> [VHAL_USSStaFCL_flg]
  [VHAL_PASAFCL_enum] -> Data Type Conversion14/1
  [VHAL_USSStaFLR_flg] -> Data Type Conversion31/1
  Subsystem/34(SNSRLayout) -> [VHAL_SNSRLayout_enum]
  Subsystem/29(USSStaFLL) -> [VHAL_USSStaFLL_flg]
  Subsystem/21(USSStaFCR) -> [VHAL_USSStaFCR_flg]
  [VHAL_PASDRCL_cm] -> Data Type Conversion2/1
  Data Type Conversion14/1 -> Bus Creator/13  "VHAL_PASAFCL_enum"
  Subsystem/1(PASDFCR) -> [VHAL_PASDFCR_cm]
  Data Type Conversion7/1 -> Bus Creator/7  "VHAL_PASDFCR_cm"
  Subsystem/2(PASDFMR) -> [VHAL_PASDFMR_cm]
  Subsystem/30(USSStaRLL) -> [VHAL_USSStaRLL_flg]
  Data Type Conversion17/1 -> Bus Creator/18  "VHAL_PASAFMR_enum"
  [VHAL_PASARMR_enum] -> Data Type Conversion12/1
  Data Type Conversion32/1 -> Bus Creator/30  "VHAL_USSStaFLL_flg"
  Subsystem/7(PASDRML) -> [VHAL_PASDRML_cm]
  Subsystem/26(USSStaRMR) -> [VHAL_USSStaRMR_flg]
  Data Type Conversion20/1 -> Bus Creator/1  "VHAL_PASDRMR_cm"
  [VHAL_USSStaRCL_flg] -> Data Type Conversion21/1
  Subsystem/10(APSDRLL) -> [VHAL_APSDRLL_cm]
  Data Type Conversion34/1 -> Bus Creator/34  "VHAL_SNSRLayout_enum"
  [VHAL_Chime_enum] -> Data Type Conversion36/1
  Data Type Conversion18/1 -> Bus Creator/22  "VHAL_USSStaRML_flg"
  [VHAL_PASDFMR_cm] -> Data Type Conversion6/1
  Data Type Conversion31/1 -> Bus Creator/29  "VHAL_USSStaFLR_flg"
  Data Type Conversion10/1 -> Bus Creator/9  "VHAL_APSDRLR_cm"
  Data Type Conversion35/1 -> Bus Creator/36  "VHAL_ModOperation_enum"
  Subsystem/31(USSStaFLR) -> [VHAL_USSStaFLR_flg]
  Data Type Conversion8/1 -> Bus Creator/10  "VHAL_APSDRLL_cm"
  [VHAL_USSStaRML_flg] -> Data Type Conversion18/1
  Subsystem/19(PASARML) -> [VHAL_PASARML_enum]
  [VHAL_USSStaFMR_flg] -> Data Type Conversion22/1
  Subsystem/22(USSStaFMR) -> [VHAL_USSStaFMR_flg]
  Data Type Conversion25/1 -> Bus Creator/20  "VHAL_PASAFCR_enum"
  Subsystem/33(Chime) -> [VHAL_Chime_enum]
  Data Type Conversion11/1 -> Bus Creator/11  "VHAL_APSDFLR_cm"
  Data Type Conversion36/1 -> Bus Creator/33  "VHAL_Chime_enum"
  [VHAL_APSDFLR_cm] -> Data Type Conversion11/1
  Subsystem/13(PASAFCR) -> [VHAL_PASAFCR_enum]
  [VHAL_PASDFCL_cm] -> Data Type Conversion5/1
  Data Type Conversion/1 -> Bus Creator/21  "VHAL_USSStaRMR_flg"
  Data Type Conversion2/1 -> Bus Creator/4  "VHAL_PASDRCL_cm"
  [VHAL_USSStaFML_flg] -> Data Type Conversion23/1
  Data Type Conversion1/1 -> Bus Creator/2  "VHAL_PASDRML_cm"
  [VHAL_USSStaRCR_flg] -> Data Type Conversion19/1
  Subsystem/25(USSStaRCR) -> [VHAL_USSStaRCR_flg]
  Subsystem/28(USSStaRCL) -> [VHAL_USSStaRCL_flg]
  [VHAL_ModOperation_enum] -> Data Type Conversion35/1
  Data Type Conversion19/1 -> Bus Creator/25  "VHAL_USSStaRCR_flg"
  Subsystem/5(PASDRCR) -> [VHAL_PASDRCR_cm]
  Data Type Conversion26/1 -> Bus Creator/17  "VHAL_PASARCL_enum"
  Data Type Conversion27/1 -> Bus Creator/19  "VHAL_PASAFML_enum"
  Subsystem/23(USSStaFML) -> [VHAL_USSStaFML_flg]
  Subsystem/17(PASARCR) -> [VHAL_PASARCR_enum]
  [VHAL_APSDRLL_cm] -> Data Type Conversion8/1
  Subsystem/6(PASDRMR) -> [VHAL_PASDRMR_cm]
  Data Type Conversion21/1 -> Bus Creator/26  "VHAL_USSStaRCL_flg"
  Data Type Conversion24/1 -> Bus Creator/31  "VHAL_USSStaFCR_flg"
  Data Type Conversion23/1 -> Bus Creator/28  "VHAL_USSStaFML_flg"
  Data Type Conversion5/1 -> Bus Creator/8  "VHAL_PASDFCL_cm"
  [VHAL_PASAFCR_enum] -> Data Type Conversion25/1
  [VHAL_PASDFCR_cm] -> Data Type Conversion7/1
  Data Type Conversion29/1 -> Bus Creator/23  "VHAL_USSStaRLR_flg"
  [VHAL_USSStaRLR_flg] -> Data Type Conversion29/1
  Subsystem/14(PASAFMR) -> [VHAL_PASAFMR_enum]
  Data Type Conversion30/1 -> Bus Creator/24  "VHAL_USSStaRLL_flg"
  Subsystem/32(USSStaRLR) -> [VHAL_USSStaRLR_flg]
  [VHAL_PASAFML_enum] -> Data Type Conversion27/1
  Data Type Conversion22/1 -> Bus Creator/27  "VHAL_USSStaFMR_flg"
  APSDistanceData/1 -> Subsystem/2(APSDistanceData)
  APSFaultStaData/1 -> Subsystem/4(APSFaultStaData)
  APSLevelData/1 -> Subsystem/3(APSLevelData)
  ChimeIn/1 -> Subsystem/5(ChimeIn)
  SNSRLayoutIn/1 -> Subsystem/6(SNSRLayoutIn)
  StaFSyaIn/1 -> Subsystem/7(StaFSyaIn)
  ModOperationIn/1 -> Subsystem/8(ModOperationIn)
  PASDistanceData/1 -> Subsystem/1(PASDistanceData)
  u8_GetAPS_HW_Ver/1 -> [VHAL_APSHWVer_enum]
  u8_GetAPS_Progress_PCT/1 -> [VHAL_APSProgressPCT_pct]
  u8_GetAPS_Req/1 -> [VHAL_APSReq_enum]
  u8_GetAPS_Sta_System/1 -> [VHAL_APSStaSystem_enum]
  u8_GetAPS_SW_Ver/1 -> [VHAL_APSSWVer_enum]
  u8_GetAPS_V_Rq_EPAS_Ctrl/1 -> [VHAL_APSVRqEPASCtrl_flg]
  u8_GetAPS_ExitCondition/1 -> [VHAL_APSExitCondition_enum]
  u8_GetCAAS_Sta/1 -> [VHAL_CAASSta_enum]
  u8_GetAPS_VMC_Req_A/1 -> [VHAL_APSVMCReqA_flg]
  f32_GetAPS_SpeedCmd/1 -> [VHAL_APSSpeedCMD_kph]
  u8_GetAPS_Rq_EPAS_Ctrl/1 -> [VHAL_APSRqEPASCtrl_flg]
  u8_GetAPS_ShftPosnReq/1 -> [VHAL_APSShiftPosnReq_enum]
  u8_GetAPS_DecReq_A/1 -> [VHAL_APSDecReqA_flg]
  f32_GetAPS_Angle_Target/1 -> [VHAL_APSAngleTarget_Deg]
  u8_GetAPS_RQ_Display/1 -> [VHAL_APSRQDisplay_enum]
  f32_GetAPS_DecReq/1 -> [VHAL_APSDecReq_mps2]
  u8_GetCAAS_VMC_Req_A/1 -> [VHAL_CAASVMCReqA_flg]
  Data Type Conversion47/1 -> Bus Creator/44  "VHAL_APSVRqEPASCtrl_flg"
  Data Type Conversion50/1 -> Bus Creator/47  "VHAL_APSDecReq_mps2"
  Data Type Conversion39/1 -> Bus Creator/50  "VHAL_APSSpeedCMD_kph"
  Data Type Conversion43/1 -> Bus Creator/40  "VHAL_APSHWVer_enum"
  Data Type Conversion38/1 -> Bus Creator/49  "VHAL_APSShiftPosnReq_enum"
  Data Type Conversion42/1 -> Bus Creator/39  "VHAL_APSSWVer_enum"
  [VHAL_APSVRqEPASCtrl_flg] -> Data Type Conversion47/1
  Data Type Conversion51/1 -> Bus Creator/48  "VHAL_APSDecReqA_flg"
  Data Type Conversion46/1 -> Bus Creator/43  "VHAL_APSStaSystem_enum"
  Data Type Conversion44/1 -> Bus Creator/41  "VHAL_APSExitCondition_enum"
  [VHAL_APSVMCReqA_flg] -> Data Type Conversion37/1
  [VHAL_APSReq_enum] -> Data Type Conversion49/1
  [VHAL_APSSpeedCMD_kph] -> Data Type Conversion39/1
  Data Type Conversion48/1 -> Bus Creator/45  "VHAL_APSRqEPASCtrl_flg"
  [VHAL_APSShiftPosnReq_enum] -> Data Type Conversion38/1
  Data Type Conversion52/1 -> Bus Creator/52  "VHAL_CAASSta_enum"
  Data Type Conversion45/1 -> Bus Creator/42  "VHAL_APSAngleTarget_Deg"
  Data Type Conversion49/1 -> Bus Creator/46  "VHAL_APSReq_enum"
  [VHAL_CAASSta_enum] -> Data Type Conversion52/1
  [VHAL_APSRqEPASCtrl_flg] -> Data Type Conversion48/1
  [VHAL_APSStaSystem_enum] -> Data Type Conversion46/1
  Data Type Conversion40/1 -> Bus Creator/37  "VHAL_APSProgressPCT_pct"
  [VHAL_APSExitCondition_enum] -> Data Type Conversion44/1
  [VHAL_APSSWVer_enum] -> Data Type Conversion42/1
  [VHAL_APSHWVer_enum] -> Data Type Conversion43/1
  [VHAL_APSAngleTarget_Deg] -> Data Type Conversion45/1
  [VHAL_APSDecReq_mps2] -> Data Type Conversion50/1
  [VHAL_APSProgressPCT_pct] -> Data Type Conversion40/1
  [VHAL_APSDecReqA_flg] -> Data Type Conversion51/1
  [VHAL_APSRQDisplay_enum] -> Data Type Conversion41/1
  Data Type Conversion41/1 -> Bus Creator/38  "VHAL_APSRQDisplay_enum"
  Data Type Conversion37/1 -> Bus Creator/51  "VHAL_APSVMCReqA_flg"
  [VHAL_CAASVMCReqA_flg] -> Data Type Conversion16/1
  Data Type Conversion16/1 -> Bus Creator/53  "VHAL_CAASVMCReqA_flg"
  u8_GetRAPS_BCM_LockReq_Cmd/1 -> [VHAL_RAPSBCMLockReq_flg]
  u8_GetRAPS_BCM_Lamp_Cmd/1 -> [VHAL_RAPSBCMLamp_enum]
  u8_GetAPS_PwrReq_cmd/1 -> [VHAL_APSPwrReq_enum]
  u8_GetRAPS_ErrWarn_Sta/1 -> [VHAL_RAPSErrWarnSta_enum]
  u8_GetRAPS_ErrLv1_flg/1 -> [VHAL_RAPSErrLv1_flg]
  [VHAL_APSPwrReq_enum] -> Data Type Conversion53/1
  [VHAL_RAPSBCMLockReq_flg] -> Data Type Conversion55/1
  [VHAL_RAPSBCMLamp_enum] -> Data Type Conversion54/1
  Data Type Conversion54/1 -> Bus Creator/56  "VHAL_RAPSBCMLamp_enum"
  Data Type Conversion55/1 -> Bus Creator/55  "VHAL_RAPSBCMLockReq_flg"
  Data Type Conversion53/1 -> Bus Creator/54  "VHAL_APSPwrReq_enum"
  [VHAL_RAPSErrWarnSta_enum] -> Data Type Conversion56/1
  [VHAL_RAPSErrLv1_flg] -> Data Type Conversion57/1
  Data Type Conversion57/1 -> Bus Creator/58  "VHAL_RAPSErrLv1_flg"
  Data Type Conversion56/1 -> Bus Creator/57  "VHAL_RAPSErrWarnSta_enum"
